simulink model "bandstop"  (Simulink 6.6)
settings: Solver=VariableStepDiscrete  StartTime=0.0  StopTime=12  RelTol=1e-3
PreLoadFcn:
  | Tsysclk=1/24000000;
  | audio_data = wavread('Yabu_sample_16_mono.wav');
  | audio_size = size(audio_data);
  | audio_time=(1:1:audio_size(1));
  | audio_in = [audio_time' audio_data];
StartFcn:
  | tic
StopFcn:
  | toc
libraries: dspbuff3 x2, simulink x2, dspwin32 x2, dspsigops x1, dsparch4 x1
settings Model: Creator=lcrockett  LastModifiedBy=lcrockett
settings OptimizationCC: InlineParams=on  InlineInvariantSignals=on
settings DebuggingCC: SignalResolutionControl=TryResolveAllWithWarning  MultiTaskDSMMsg=warning  MultiTaskCondExecSysMsg=none  StrictBusMsg=None
settings HardwareCC: TargetHWDeviceType=32-bit Generic  ProdEqTarget=off
settings RTWCC: IncludeERTFirstTime=on

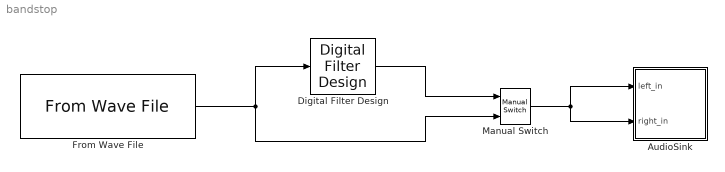
== system bandstop ==
  AudioSink : Subsystem
  Digital Filter Design : dsparch4/Digital Filter Design  SystemSampleTime=-1  mwdsp_browser_bugfix_var=off
  From Wave File : dspwin32/From Wave File  FileName=Yabu_sample_2kHz_tone  SamplesPerFrame=1  MinBufSize=1  dType=double  bLoop=off  timesToPlay=1  restartMode=immediately after last sample  firstSampleOutput=off  lastSampleOutput=off
  Manual Switch : simulink/Signal Routing/Manual Switch  SystemSampleTime=-1  sw=1  action=0  varsize=off
  wires:
  From Wave File/1 -> Digital Filter Design/1, Manual Switch/2
  Digital Filter Design/1 -> Manual Switch/1
  Manual Switch/1 -> AudioSink/1(left_in), AudioSink/2(right_in)

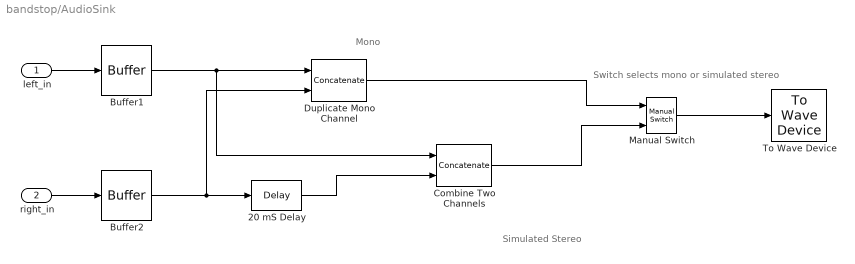
== system bandstop/AudioSink ==
  note: Mono
  note: Simulated
      | Stereo
  note: Switch selects mono
      | or simulated stereo
  left_in : Inport
  right_in : Inport  Port=2
  20 mS Delay : dspsigops/Delay  dly_unit=Samples  delay=20e-3 * 48000  ic_detail=on  dif_ic_for_ch=off  dif_ic_for_dly=off  ic=0  reset_popup=None
  Buffer1 : dspbuff3/Buffer  N=1  V=0  ic=0
  Buffer2 : dspbuff3/Buffer  N=1  V=0  ic=0
  Combine Two Channels : Concatenate  Mode=Multidimensional array  ConcatenateDimension=2
  Duplicate Mono Channel : Concatenate  Mode=Multidimensional array  ConcatenateDimension=2
  Manual Switch : simulink/Signal Routing/Manual Switch  SystemSampleTime=-1  sw=1  action=0
  To Wave Device : dspwin32/To Wave Device  bufDuration=0.1  determineBufSize=on  userIntBufSize=256  initDelay=0.1  useDefaultDevice=on  userDeviceID=SigmaTel Audio  enable24Bit=off
  wires:
  20 mS Delay/1 -> Combine Two Channels/2
  Duplicate Mono Channel/1 -> Manual Switch/1
  left_in/1 -> Buffer1/1
  Manual Switch/1 -> To Wave Device/1
  Combine Two Channels/1 -> Manual Switch/2
  right_in/1 -> Buffer2/1
  Buffer2/1 -> Duplicate Mono Channel/2, 20 mS Delay/1
  Buffer1/1 -> Duplicate Mono Channel/1, Combine Two Channels/1
